simulink model "Pacemaker_group11_requirementtable"  (R2022a)
settings: Solver=FixedStepAuto  StartTime=0.0  StopTime=10.0  FixedStep=1e-3  RelTol=1e-3  EnableMultiTasking=on
undefined symbols (not defined in the file): A0, A1, D0, D1, D10, D11, D12, D13, D2, D3, D4, D5, D6, D7, D8, D9, magnitude, PTA0, PTA1, PTA2, PTB2, PTB23, PTB3, PTB9, PTC16, PTC17, PTC2, PTC3, PTC4, PTD0, PTD1, PTD2, PTD3
libraries: frdmk64flib x20, etargetslib x17, dspstat3 x1, simulink x1
(part 2 of 2)

== stateflow chart Pacemaker_group11_requirementtable/eight model stateflow ==
  state Start
  state AOO [group]
    state Charging_C22
      entry:
      %Charging C22 and discharging C21
      PACING_REF_PWM = ATR_DUTY_CYCLE;
      PACE_CHARGE_CTRL = true;
      PACE_GND_CTRL = true;
      ATR_PACE_CTRL = false;
      Z_ATR_CTRL = false;
      Z_VENT_CTRL = false;
      VENT_PACE_CTRL = false;
      VENT_GND_CTRL = false;
      ATR_GND_CTRL = true;
      % For LED testing
      IS_CHARGING = true;
      %For requirement table
      status=00000;
    state Pacing
      entry:
      PACE_CHARGE_CTRL = false;
      PACE_GND_CTRL = true;
      VENT_PACE_CTRL = false;
      VENT_GND_CTRL = false;
      Z_ATR_CTRL = false;
      Z_VENT_CTRL = false;
      ATR_GND_CTRL = false;
      ATR_PACE_CTRL = true;
      % For LED testing
      IS_CHARGING = false;
      %For requirement table
      status=00001;
    AOO.Charging_C22 -> AOO.Pacing [order 1] : [after(PULSE_PERIOD-ATR_PW,msec)]
    AOO.Pacing -> AOO.Charging_C22 : [after(ATR_PW,msec)]
  state VOO [group]
    state Charging_C22
      entry:
      %Charging C22 and discharging C21
      PACING_REF_PWM = VENT_DUTY_CYCLE;
      PACE_CHARGE_CTRL = true;
      PACE_GND_CTRL = true;
      VENT_PACE_CTRL = false;
      Z_ATR_CTRL = false;
      Z_VENT_CTRL = false;
      ATR_PACE_CTRL = false;
      ATR_GND_CTRL = false;
      VENT_GND_CTRL = true;
      % For LED testing
      IS_CHARGING = true;
      %For requirement table
      status=00010;
    state Pacing
      entry:
      PACE_CHARGE_CTRL = false;
      PACE_GND_CTRL = true;
      ATR_PACE_CTRL = false;
      ATR_GND_CTRL = false;
      Z_ATR_CTRL = false;
      Z_VENT_CTRL = false;
      VENT_GND_CTRL = false;
      VENT_PACE_CTRL = true;
      % For LED testing
      IS_CHARGING = false;
      %For requirement table
      status=00011;
    VOO.Charging_C22 -> VOO.Pacing [order 1] : [after(PULSE_PERIOD-VENT_PW,msec)]
    VOO.Pacing -> VOO.Charging_C22 : [after(VENT_PW,msec)]
  state AAI [group]
    state Charging_C22
      entry:
      %Charging C22 and discharging C21
      PACING_REF_PWM = ATR_DUTY_CYCLE;
      PACE_CHARGE_CTRL = true;
      PACE_GND_CTRL = true;
      ATR_PACE_CTRL = false;
      Z_ATR_CTRL = false;
      Z_VENT_CTRL = false;
      VENT_PACE_CTRL = false;
      VENT_GND_CTRL = false;
      ATR_GND_CTRL = true;
      % For LED testing
      IS_CHARGING = true;
      FRONTEND_CTRL = true;
      %For requirement table
      status=00100;
    state Proxy
      entry:
      %Charging C22 and discharging C21
      PACING_REF_PWM = ATR_DUTY_CYCLE;
      PACE_CHARGE_CTRL = true;
      PACE_GND_CTRL = true;
      ATR_PACE_CTRL = false;
      Z_ATR_CTRL = false;
      Z_VENT_CTRL = false;
      VENT_PACE_CTRL = false;
      VENT_GND_CTRL = false;
      ATR_GND_CTRL = true;
      % For LED testing
      IS_CHARGING = true;
      %For requirement table
      status=00101;
    state Pacing
      entry:
      PACE_CHARGE_CTRL = false;
      PACE_GND_CTRL = true;
      VENT_PACE_CTRL = false;
      VENT_GND_CTRL = false;
      Z_ATR_CTRL = false;
      Z_VENT_CTRL = false;
      ATR_GND_CTRL = false;
      ATR_PACE_CTRL = true;
      % For LED testing
      IS_CHARGING = false;
      %For requirement table
      status=00110;
    AAI.Charging_C22 -> AAI.Proxy [order 1] : [ATR_CMP_DETECT ==  true]{DELAY = ARP}
    AAI.Proxy -> AAI.Charging_C22 : [after(DELAY,msec)]
    AAI.Charging_C22 -> AAI.Pacing [order 2] : [after(PULSE_PERIOD-ARP,msec)]
    AAI.Pacing -> AAI.Proxy : [after(ATR_PW,msec)]{DELAY = ARP - ATR_PW }
  state VVI [group]
    state Charging_C22
      entry:
      %Charging C22 and discharging C21
      PACING_REF_PWM = VENT_DUTY_CYCLE;
      PACE_CHARGE_CTRL = true;
      PACE_GND_CTRL = true;
      VENT_PACE_CTRL = false;
      Z_ATR_CTRL = false;
      Z_VENT_CTRL = false;
      ATR_PACE_CTRL = false;
      ATR_GND_CTRL = false;
      VENT_GND_CTRL = true;
      % For LED testing
      IS_CHARGING = true;
      FRONTEND_CTRL = true;
      %For requirement table
      status=00111;
    state Proxy
      entry:
      %Charging C22 and discharging C21
      PACING_REF_PWM = VENT_DUTY_CYCLE;
      PACE_CHARGE_CTRL = true;
      PACE_GND_CTRL = true;
      VENT_PACE_CTRL = false;
      Z_ATR_CTRL = false;
      Z_VENT_CTRL = false;
      ATR_PACE_CTRL = false;
      ATR_GND_CTRL = false;
      VENT_GND_CTRL = true;
      % For LED testing
      IS_CHARGING = true;
      %For requirement table
      status=01000;
    note: %For requirement table
        | status=0000;
    state Pacing
      entry:
      PACE_CHARGE_CTRL = false;
      PACE_GND_CTRL = true;
      ATR_PACE_CTRL = false;
      ATR_GND_CTRL = false;
      Z_ATR_CTRL = false;
      Z_VENT_CTRL = false;
      VENT_GND_CTRL = false;
      VENT_PACE_CTRL = true;
      % For LED testing
      IS_CHARGING = false;
      %For requirement table
      status=01001;
    VVI.Charging_C22 -> VVI.Proxy [order 1] : [VENT_CMP_DETECT ==  true]{DELAY = VRP}
    VVI.Proxy -> VVI.Charging_C22 : [after(DELAY,msec)]
    VVI.Charging_C22 -> VVI.Pacing [order 2] : [after(PULSE_PERIOD-VRP,msec)]
    VVI.Pacing -> VVI.Proxy : [after(VENT_PW,msec)]{DELAY = VRP - VENT_PW }
  state AOOR [group]
    state Charging_C22
      entry:
      PACING_REF_PWM = ATR_DUTY_CYCLE
      PACE_CHARGE_CTRL = true
      PACE_GND_CTRL = true
      ATR_PACE_CTRL = false
      Z_ATR_CTRL = false
      Z_VENT_CTRL = false
      VENT_PACE_CTRL = false
      VENT_GND_CTRL = false
      ATR_GND_CTRL = true
      % For LED testing
      IS_CHARGING = true
    state Pacing
      entry:
      PACE_CHARGE_CTRL = false
      PACE_GND_CTRL = true
      VENT_PACE_CTRL = false
      VENT_GND_CTRL = false
      Z_ATR_CTRL = false
      Z_VENT_CTRL = false
      ATR_GND_CTRL = false
      ATR_PACE_CTRL = true
      % For LED testing
      IS_CHARGING = false
    AOOR.Charging_C22 -> AOOR.Pacing [order 1] : [after(MODIFIED_PERIOD-ATR_PW,msec)]
    AOOR.Pacing -> AOOR.Charging_C22 : [after(ATR_PW,msec)]
  state VOOR [group]
    state Charging_C22
      entry:
      PACING_REF_PWM = VENT_DUTY_CYCLE
      PACE_CHARGE_CTRL = true
      PACE_GND_CTRL = true
      VENT_PACE_CTRL = false
      Z_ATR_CTRL = false
      Z_VENT_CTRL = false
      ATR_PACE_CTRL = false
      ATR_GND_CTRL = false
      VENT_GND_CTRL = true
      % For LED testing
      IS_CHARGING = true
    state Pacing
      entry:
      PACE_CHARGE_CTRL = false
      PACE_GND_CTRL = true
      ATR_PACE_CTRL = false
      ATR_GND_CTRL = false
      Z_ATR_CTRL = false
      Z_VENT_CTRL = false
      VENT_GND_CTRL = false
      VENT_PACE_CTRL = true
      % For LED testing
      IS_CHARGING = false
    VOOR.Charging_C22 -> VOOR.Pacing [order 1] : [after(MODIFIED_PERIOD-VENT_PW,msec)]
    VOOR.Pacing -> VOOR.Charging_C22 : [after(VENT_PW,msec)]
  state AAIR [group]
    state Charging_C22
      entry:
      PACING_REF_PWM = ATR_DUTY_CYCLE;
      PACE_CHARGE_CTRL = true;
      PACE_GND_CTRL = true;
      ATR_PACE_CTRL = false;
      Z_ATR_CTRL = false;
      Z_VENT_CTRL = false;
      VENT_PACE_CTRL = false;
      VENT_GND_CTRL = false;
      ATR_GND_CTRL = true;
      % For LED testing
      IS_CHARGING = true;
      FRONTEND_CTRL = true;
      %For requirement table
      status=01110;
    state Proxy
      entry:
      PACING_REF_PWM = ATR_DUTY_CYCLE;
      PACE_CHARGE_CTRL = true;
      PACE_GND_CTRL = true;
      ATR_PACE_CTRL = false;
      Z_ATR_CTRL = false;
      Z_VENT_CTRL = false;
      VENT_PACE_CTRL = false;
      VENT_GND_CTRL = false;
      ATR_GND_CTRL = true;
      % For LED testing
      IS_CHARGING = true;
      %For requirement table
      status=01111;
    state Pacing
      entry:
      PACE_CHARGE_CTRL = false;
      PACE_GND_CTRL = true;
      VENT_PACE_CTRL = false;
      VENT_GND_CTRL = false;
      Z_ATR_CTRL = false;
      Z_VENT_CTRL = false;
      ATR_GND_CTRL = false;
      ATR_PACE_CTRL = true;
      % For LED testing
      IS_CHARGING = false;
      %For requirement table
      status=10000;
    AAIR.Charging_C22 -> AAIR.Proxy [order 1] : [ATR_CMP_DETECT ==  true]{DELAY = ARP}
    AAIR.Proxy -> AAIR.Charging_C22 : [after(DELAY,msec)]
    AAIR.Charging_C22 -> AAIR.Pacing [order 2] : [after(MODIFIED_PERIOD-ARP,msec)]
    AAIR.Pacing -> AAIR.Proxy : [after(ATR_PW,msec)]{DELAY = ARP - ATR_PW }
  state VVIR [group]
    state Charging_C22
      entry:
      PACING_REF_PWM = VENT_DUTY_CYCLE;
      PACE_CHARGE_CTRL = true;
      PACE_GND_CTRL = true;
      VENT_PACE_CTRL = false;
      Z_ATR_CTRL = false;
      Z_VENT_CTRL = false;
      ATR_PACE_CTRL = false;
      ATR_GND_CTRL = false;
      VENT_GND_CTRL = true;
      % For LED testing
      IS_CHARGING = true;
      FRONTEND_CTRL = true;
      %For requirement table
      status=10001;
    state Proxy
      entry:
      PACING_REF_PWM = VENT_DUTY_CYCLE;
      PACE_CHARGE_CTRL = true;
      PACE_GND_CTRL = true;
      VENT_PACE_CTRL = false;
      Z_ATR_CTRL = false;
      Z_VENT_CTRL = false;
      ATR_PACE_CTRL = false;
      ATR_GND_CTRL = false;
      VENT_GND_CTRL = true;
      % For LED testing
      IS_CHARGING = true;
      %For requirement table
      status=10010;
    state Pacing
      entry:
      PACE_CHARGE_CTRL = false;
      PACE_GND_CTRL = true;
      ATR_PACE_CTRL = false;
      ATR_GND_CTRL = false;
      Z_ATR_CTRL = false;
      Z_VENT_CTRL = false;
      VENT_GND_CTRL = false;
      VENT_PACE_CTRL = true;
      % For LED testing
      IS_CHARGING = false;
      %For requirement table
      status=10011;
    VVIR.Charging_C22 -> VVIR.Proxy [order 1] : [VENT_CMP_DETECT ==  true]{DELAY = VRP}
    VVIR.Proxy -> VVIR.Charging_C22 : [after(DELAY,msec)]
    VVIR.Charging_C22 -> VVIR.Pacing [order 2] : [after(MODIFIED_PERIOD-VRP,msec)]
    VVIR.Pacing -> VVIR.Proxy : [after(VENT_PW,msec)]{DELAY = VRP - VENT_PW }
  VOOR.Charging_C22 -> Start [order 2] : [MODE ~= 6]
  VVIR.Charging_C22 -> Start [order 3] : [MODE ~= 8]
  AAIR.Charging_C22 -> Start [order 3] : [MODE ~= 7]
  Start -> AOO.Charging_C22 [order 2] : [MODE == 1]
  Start -> VOO.Charging_C22 [order 1] : [MODE == 2]
  AOOR.Charging_C22 -> Start [order 2] : [MODE ~= 5]
  Start -> VVI.Charging_C22 [order 7] : [MODE == 4]
  Start -> AOOR.Charging_C22 [order 4] : [MODE == 5]
  (default) -> Start
  Start -> VOOR.Charging_C22 [order 8] : [MODE == 6]
  VVI.Charging_C22 -> Start [order 3] : [MODE ~= 4]
  Start -> AAI.Charging_C22 [order 3] : [MODE == 3]
  AAI.Charging_C22 -> Start [order 3] : [MODE ~= 3]
  AOO.Charging_C22 -> Start [order 2] : [MODE ~= 1]
  VOO.Charging_C22 -> Start [order 2] : [MODE ~= 2]
  Start -> AAIR.Charging_C22 [order 5] : [MODE == 7]
  Start -> VVIR.Charging_C22 [order 6] : [MODE == 8]
  data: IS_CHARGING output; PACE_CHARGE_CTRL output; Z_ATR_CTRL output; PACING_REF_PWM output; Z_VENT_CTRL output; ATR_PACE_CTRL output; VENT_PACE_CTRL output; PACE_GND_CTRL output; ATR_GND_CTRL output; VENT_GND_CTRL output; FRONTEND_CTRL output =true; VENT_DUTY_CYCLE input; PULSE_PERIOD input; VENT_CMP_DETECT input; DELAY local; ATR_DUTY_CYCLE input; ATR_CMP_DETECT input; MODIFIED_PERIOD input; MODE input; ATR_PW input; VENT_PW input; VRP input; ARP input; status output

== stateflow chart Pacemaker_group11_requirementtable/get desired rate ==
  state check
    %check if the actvity level below the threshold
  state Desires_output_1
    entry:
    DESIRED_RATE=LRL;
  state Desires_output_3
    entry:
    DESIRED_RATE = Local_rate;
  state Desires_output_2
    entry:
    DESIRED_RATE = MSR;
  state Increase_Linear
    entry:
    Local_rate = LRL + RESPONSE_FACTOR*(ACTIVITY_LEVEL-ACTIVITY_THRESHOLD);
  (default) -> check
  check -> Desires_output_1 [order 1] : [ACTIVITY_LEVEL<=ACTIVITY_THRESHOLD]
  Desires_output_1 -> check : after(100,msec)
  check -> Increase_Linear [order 2] : [ACTIVITY_LEVEL>ACTIVITY_THRESHOLD]
  Desires_output_3 -> check : after(100,msec)
  Desires_output_2 -> check : after(100,msec)
  Increase_Linear -> Desires_output_2 [order 1] : [Local_rate >=MSR]
  Increase_Linear -> Desires_output_3 [order 2] : [Local_rate<MSR]
  data: ACTIVITY_LEVEL input; LRL input; MSR input; ACTIVITY_THRESHOLD input; RESPONSE_FACTOR input; DESIRED_RATE output; Local_rate local

== stateflow chart Pacemaker_group11_requirementtable/get target rate ==
  state increase_state
    entry:
    %use linear:
    if(Target_rate<MSR && Target_rate<DESIRED_RATE)
    Target_rate=Target_rate+step_up;
    elseif(Target_rate == DESIRED_RATE)
    Target_rate = DESIRED_RATE;
    elseif(Target_rate>MSR)
    Target_rate = MSR
    end
  state step_state
    entry:
    step_up = (MSR-LRL)/REACTION_TIME;
    step_down = (MSR-LRL)/RECOVER_TIME;
  state decrease_state
    entry:
    if(Target_rate<MSR)
    Target_rate = Target_rate - step_down;
    elseif(Target_rate <= LRL)
    Target_rate = LRL;
    end
  state start_state
    %set target rate to at least LRL
    Target_rate = LRL;
  step_state -> increase_state [order 2] : after(100,msec)[Target_rate<=DESIRED_RATE]
  increase_state -> step_state : after(100,msec)
  (default) -> start_state
  step_state -> decrease_state [order 1] : after(100,msec)[Target_rate>DESIRED_RATE]
  decrease_state -> step_state : after(100,msec)
  start_state -> step_state : [Target_rate>=LRL]
  data: DESIRED_RATE input; Target_rate output; LRL input; MSR input; REACTION_TIME input; RECOVER_TIME input; step_down local; step_up local
